simulink model "task2_x_func"  (R2021b)
settings: Solver=FixedStepAuto  StartTime=0.0  StopTime=3  FixedStep=0.0001  RelTol=1e-3
settings Model: Creator=den  LastModifiedBy=den

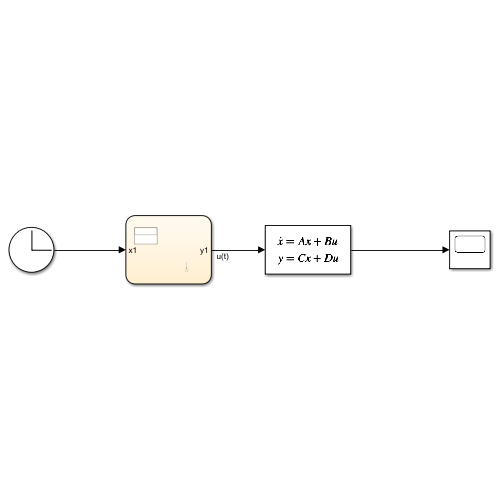
[thumbnail: Simulink's stored preview of the top-level diagram]
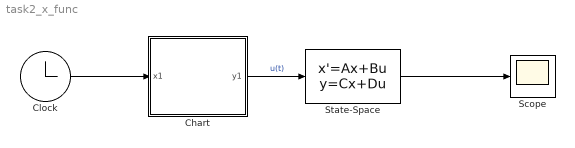
== system task2_x_func ==
  Chart : Stateflow chart  TreatAsAtomicUnit=on
  Clock : Clock
  Scope : Scope
  State-Space : StateSpace  A=[5 -2 8; 4 -3 4; -4 0 -7]  B=[-1; -3; 3]  C=[1 0 0; 0 1 0; 0 0 1]  D=[0; 0; 0]  InitialCondition=0
  wires:
  Clock/1 -> Chart/1(x1)
  Chart/1(y1) -> State-Space/1  "u(t)"
  State-Space/1 -> Scope/1

== matlab function task2_x_func/Chart ==
  data: x function_input; y function_output; x1 input; y1 output
function y = u(x)
    y = (2.7183 .^ x) .* (0.16191 .* cos(6 - 2 .* x) - 0.10679 .* sin(6 - 2 .* x));
end
